simulink model "p1a4"  (R2023b)
settings: Solver=VariableStepAuto  StartTime=0.0  StopTime=5  RelTol=1e-3
settings Model: Creator=tanvi  LastModifiedBy=m96sz

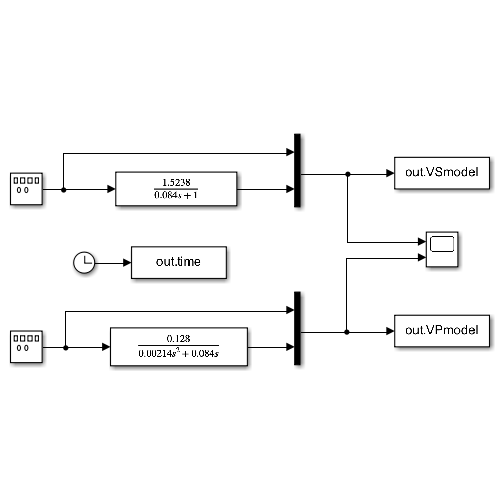
[thumbnail: Simulink's stored preview of the top-level diagram]
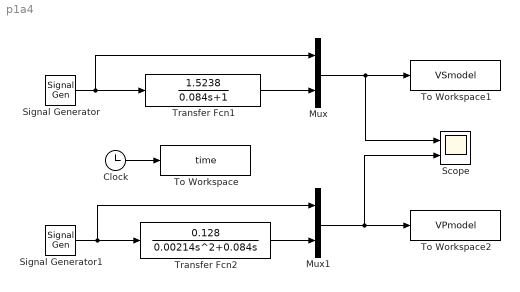
== system p1a4 ==
  Clock : Clock
      settings: Decimation=100
  Mux : Mux  Inputs=2
  Mux1 : Mux  Inputs=2
  Scope : Scope  NumInputPorts=2
  Signal Generator : SignalGenerator  WaveForm=square  Frequency=0.5
  Signal Generator1 : SignalGenerator  WaveForm=square  Frequency=0.5
  To Workspace : ToWorkspace  VariableName=time  SampleTime=-1
  To Workspace1 : ToWorkspace  VariableName=VSmodel  SampleTime=-1
  To Workspace2 : ToWorkspace  VariableName=VPmodel  SampleTime=-1
  Transfer Fcn1 : TransferFcn  Numerator=[1.5238]  Denominator=[0.084 1]
  Transfer Fcn2 : TransferFcn  Numerator=[0.128]  Denominator=[0.00214 0.084 0]
  wires:
  Signal Generator1/1 -> Transfer Fcn2/1, Mux1/1
  Clock/1 -> To Workspace/1
  Signal Generator/1 -> Mux/1, Transfer Fcn1/1
  Transfer Fcn2/1 -> Mux1/2
  Transfer Fcn1/1 -> Mux/2
  Mux/1 -> Scope/1, To Workspace1/1
  Mux1/1 -> To Workspace2/1, Scope/2
